simulink subsystem "InVoltage_to_AnchorCurrent"  (R2023a)
settings: Solver=VariableStepAuto  StartTime=0.0  StopTime=10.0  RelTol=1e-3
model mask{R_a=R_a, L_a=L_a, L_ew=L_ew}
  mask prompts: R_a "Anchor res"; L_a "Anchor inductivity"; L_ew "Inductivity of EW"
settings Model: Creator=ПК  LastModifiedBy=ПК

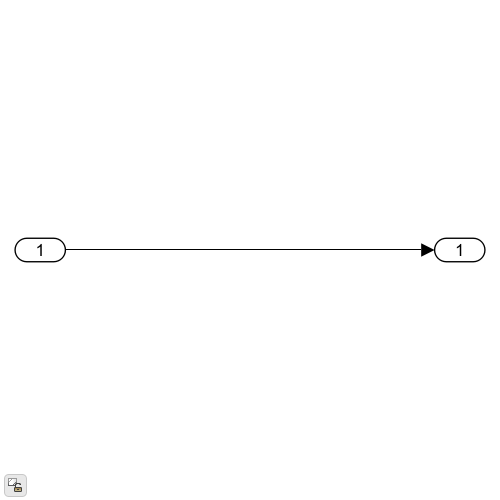
[thumbnail: Simulink's stored preview of the top-level diagram]
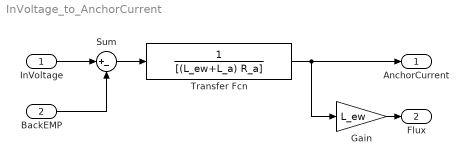
== system InVoltage_to_AnchorCurrent ==
  InVoltage : Inport
  BackEMP : Inport  Port=2
  Gain : Gain  Gain=L_ew
  Sum : Sum  Inputs=|+-
  Transfer Fcn : TransferFcn  Denominator=[(L_ew+L_a) R_a]
  AnchorCurrent : Outport
  Flux : Outport  Port=2
  wires:
  InVoltage/1 -> Sum/1
  BackEMP/1 -> Sum/2
  Sum/1 -> Transfer Fcn/1
  Transfer Fcn/1 -> AnchorCurrent/1, Gain/1
  Gain/1 -> Flux/1
